simulink model "KalmanFilterBasic"  (R2020a)
settings: Solver=VariableStepAuto  StartTime=0.0  StopTime=10  RelTol=1e-3
PostLoadFcn:
  | cd 'C:\Users\rag\Documents\GitHub\EPQ\Rocket'
  | masscgI = xlsread('mass,cg,I','mass,cg,I');
  | ThrustTable = xlsread('F10_Thrust','Sheet1');
values from neighbouring files (symbols this model uses):
  D = zeros(size(B))    [RocketOutputFunction.m]    (also in StateSpaceController.m = zeros(13, 3); TimeDelayCompensationElevator.m = [0; 0])
undefined symbols (not defined in the file or in its folder): e0_0, e1_0, e2_0, e3_0
libraries: sharedTrackingLibrary x5, aerolibcommonsys x4, shared6dof x4, sharedtransform x3, shared6dofsys x2, dspmtrx3 x1, mspsensorlib x1, simulink x1, sharedutil x1, aerolibnav x1, dspstat3 x1
settings Model: Creator=rag  LastModifiedBy=rag
settings SFSimCC: CustomCodeUndefinedFunction=UseInterfaceOnly

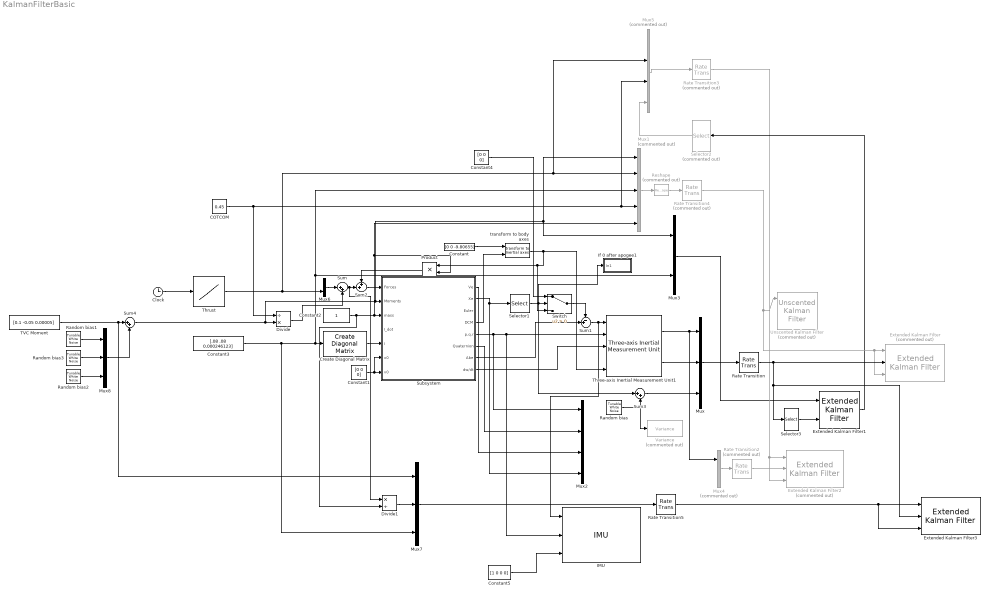
== system KalmanFilterBasic ==
  COTCOM : Constant  Value=0.45
  Clock : Clock
      settings: Decimation=100
  Constant : Constant  Value=[0 0 -9.80655]
  Constant1 : Constant  Value=[0 0 0]
  Constant2 : Constant
  Constant3 : Constant  Value=[.08 .08 0.000246123]
  Constant4 : Constant  Value=[0 0 0]
  Constant5 : Constant  Value=[1 0 0 0]
  Create Diagonal Matrix : dspmtrx3/Create Diagonal Matrix
      settings: SourceProductBaseCode=DS
  Divide : Product  Inputs=/*
  Divide1 : Product  Inputs=*/
  Extended Kalman Filter : sharedTrackingLibrary/Extended Kalman Filter  Commented=on  StateTransitionFcn=vdpStateFcn  HasStateTransitionJacobianFcn=off  HasAdditiveProcessNoise=Nonadditive  ProcessNoise=0.001 * eye(3)  HasTimeVaryingProcessNoise=off  HasStateTransitionFcnExtraArgument=1  InitialState=[zeros(1, 3) 1 zeros(1, 9)]  InitialStateCovariance=0.0000000001  MeasurementFcn1=vdpMeasurementNonAdditiveNoiseFcn  HasMeasurementJacobianFcn1=off  HasMeasurementEnablePort1=off  HasAdditiveMeasurementNoise1=Nonadditive  MeasurementNoise1=diag([0.001/0.001 0.001/0.001 0.001/0.001])  HasTimeVaryingMeasurementNoise1=off  HasMeasurementFcnExtraArgument1=1  MeasurementFcn2=myMeasurementFcn  HasMeasurementJacobianFcn2=off  HasMeasurementEnablePort2=off  HasAdditiveMeasurementNoise2=Additive  MeasurementNoise2=1  HasTimeVaryingMeasurementNoise2=off  HasMeasurementFcnExtraArgument2=0  MeasurementFcn3=myMeasurementFcn  HasMeasurementJacobianFcn3=off  HasMeasurementEnablePort3=off  HasAdditiveMeasurementNoise3=Additive  MeasurementNoise3=1  HasTimeVaryingMeasurementNoise3=off  HasMeasurementFcnExtraArgument3=0  MeasurementFcn4=myMeasurementFcn  HasMeasurementJacobianFcn4=off  HasMeasurementEnablePort4=off  HasAdditiveMeasurementNoise4=Additive  MeasurementNoise4=1  HasTimeVaryingMeasurementNoise4=off  HasMeasurementFcnExtraArgument4=0  MeasurementFcn5=myMeasurementFcn  HasMeasurementJacobianFcn5=off  HasMeasurementEnablePort5=off  HasAdditiveMeasurementNoise5=Additive  MeasurementNoise5=1  HasTimeVaryingMeasurementNoise5=off  HasMeasurementFcnExtraArgument5=0  EnableMultirate=off  StateTransitionFcnSampleTime=1  MeasurementFcn1SampleTime=1  MeasurementFcn2SampleTime=1  MeasurementFcn3SampleTime=1  MeasurementFcn4SampleTime=1  MeasurementFcn5SampleTime=1  UseCurrentEstimator=on  OutputStateCovariance=off  DataType=double  SampleTime=.2  NumberOfMeasurements=1
      settings: SourceProductBaseCode=CT,DR,TF,ID,NV,AR,RO,VE
  Extended Kalman Filter1 : sharedTrackingLibrary/Extended Kalman Filter  StateTransitionFcn=vdpStateFcnAttitudeOnly  HasStateTransitionJacobianFcn=off  HasAdditiveProcessNoise=Nonadditive  ProcessNoise=[1 1 0.001]  HasTimeVaryingProcessNoise=off  HasStateTransitionFcnExtraArgument=1  InitialState=[0 0 0 1 0 0 0]  InitialStateCovariance=1e-7  MeasurementFcn1=vdpMeasurementNonAdditiveNoiseFcnAttitudeOnly  HasMeasurementJacobianFcn1=off  HasMeasurementEnablePort1=off  HasAdditiveMeasurementNoise1=Nonadditive  MeasurementNoise1=1e-3 * eye(3)  HasTimeVaryingMeasurementNoise1=off  HasMeasurementFcnExtraArgument1=0  MeasurementFcn2=myMeasurementFcn  HasMeasurementJacobianFcn2=off  HasMeasurementEnablePort2=off  HasAdditiveMeasurementNoise2=Additive  MeasurementNoise2=1  HasTimeVaryingMeasurementNoise2=off  HasMeasurementFcnExtraArgument2=0  MeasurementFcn3=myMeasurementFcn  HasMeasurementJacobianFcn3=off  HasMeasurementEnablePort3=off  HasAdditiveMeasurementNoise3=Additive  MeasurementNoise3=1  HasTimeVaryingMeasurementNoise3=off  HasMeasurementFcnExtraArgument3=0  MeasurementFcn4=myMeasurementFcn  HasMeasurementJacobianFcn4=off  HasMeasurementEnablePort4=off  HasAdditiveMeasurementNoise4=Additive  MeasurementNoise4=1  HasTimeVaryingMeasurementNoise4=off  HasMeasurementFcnExtraArgument4=0  MeasurementFcn5=myMeasurementFcn  HasMeasurementJacobianFcn5=off  HasMeasurementEnablePort5=off  HasAdditiveMeasurementNoise5=Additive  MeasurementNoise5=1  HasTimeVaryingMeasurementNoise5=off  HasMeasurementFcnExtraArgument5=0  EnableMultirate=off  StateTransitionFcnSampleTime=1  MeasurementFcn1SampleTime=1  MeasurementFcn2SampleTime=1  MeasurementFcn3SampleTime=1  MeasurementFcn4SampleTime=1  MeasurementFcn5SampleTime=1  UseCurrentEstimator=on  OutputStateCovariance=off  DataType=double  SampleTime=0.001  NumberOfMeasurements=1
      settings: SourceProductBaseCode=CT,DR,TF,ID,NV,AR,RO,VE
  Extended Kalman Filter2 : sharedTrackingLibrary/Extended Kalman Filter  Commented=on  StateTransitionFcn=vdpStateFcnTranslationOnly  HasStateTransitionJacobianFcn=off  HasAdditiveProcessNoise=Nonadditive  ProcessNoise=0.001 * eye(3)  HasTimeVaryingProcessNoise=off  HasStateTransitionFcnExtraArgument=1  InitialState=[0 0 0 0 0 0]  InitialStateCovariance=1  MeasurementFcn1=vdpMeasurementNonAdditiveNoiseFcnTranslationOnly  HasMeasurementJacobianFcn1=off  HasMeasurementEnablePort1=off  HasAdditiveMeasurementNoise1=Nonadditive  MeasurementNoise1=diag([2 2 2 5])  HasTimeVaryingMeasurementNoise1=off  HasMeasurementFcnExtraArgument1=1  MeasurementFcn2=myMeasurementFcn  HasMeasurementJacobianFcn2=off  HasMeasurementEnablePort2=off  HasAdditiveMeasurementNoise2=Additive  MeasurementNoise2=1  HasTimeVaryingMeasurementNoise2=off  HasMeasurementFcnExtraArgument2=0  MeasurementFcn3=myMeasurementFcn  HasMeasurementJacobianFcn3=off  HasMeasurementEnablePort3=off  HasAdditiveMeasurementNoise3=Additive  MeasurementNoise3=1  HasTimeVaryingMeasurementNoise3=off  HasMeasurementFcnExtraArgument3=0  MeasurementFcn4=myMeasurementFcn  HasMeasurementJacobianFcn4=off  HasMeasurementEnablePort4=off  HasAdditiveMeasurementNoise4=Additive  MeasurementNoise4=1  HasTimeVaryingMeasurementNoise4=off  HasMeasurementFcnExtraArgument4=0  MeasurementFcn5=myMeasurementFcn  HasMeasurementJacobianFcn5=off  HasMeasurementEnablePort5=off  HasAdditiveMeasurementNoise5=Additive  MeasurementNoise5=1  HasTimeVaryingMeasurementNoise5=off  HasMeasurementFcnExtraArgument5=0  EnableMultirate=off  StateTransitionFcnSampleTime=1  MeasurementFcn1SampleTime=1  MeasurementFcn2SampleTime=1  MeasurementFcn3SampleTime=1  MeasurementFcn4SampleTime=1  MeasurementFcn5SampleTime=1  UseCurrentEstimator=on  OutputStateCovariance=off  DataType=double  SampleTime=0.001  NumberOfMeasurements=1
      settings: SourceProductBaseCode=CT,DR,TF,ID,NV,AR,RO,VE
  Extended Kalman Filter3 : sharedTrackingLibrary/Extended Kalman Filter  StateTransitionFcn=vdpStateFcn  HasStateTransitionJacobianFcn=off  HasAdditiveProcessNoise=Nonadditive  ProcessNoise=[.1 .1 1e-5]  HasTimeVaryingProcessNoise=off  HasStateTransitionFcnExtraArgument=1  InitialState=[zeros(1,3) 1 zeros(1,9)]  InitialStateCovariance=1e-9  MeasurementFcn1=vdpMeasurementNonAdditiveNoiseFcn  HasMeasurementJacobianFcn1=off  HasMeasurementEnablePort1=off  HasAdditiveMeasurementNoise1=Nonadditive  MeasurementNoise1=diag([.1 .1 .1 .1 .1 .1 1])  HasTimeVaryingMeasurementNoise1=off  HasMeasurementFcnExtraArgument1=1  MeasurementFcn2=myMeasurementFcn  HasMeasurementJacobianFcn2=off  HasMeasurementEnablePort2=off  HasAdditiveMeasurementNoise2=Additive  MeasurementNoise2=1  HasTimeVaryingMeasurementNoise2=off  HasMeasurementFcnExtraArgument2=0  MeasurementFcn3=myMeasurementFcn  HasMeasurementJacobianFcn3=off  HasMeasurementEnablePort3=off  HasAdditiveMeasurementNoise3=Additive  MeasurementNoise3=1  HasTimeVaryingMeasurementNoise3=off  HasMeasurementFcnExtraArgument3=0  MeasurementFcn4=myMeasurementFcn  HasMeasurementJacobianFcn4=off  HasMeasurementEnablePort4=off  HasAdditiveMeasurementNoise4=Additive  MeasurementNoise4=1  HasTimeVaryingMeasurementNoise4=off  HasMeasurementFcnExtraArgument4=0  MeasurementFcn5=myMeasurementFcn  HasMeasurementJacobianFcn5=off  HasMeasurementEnablePort5=off  HasAdditiveMeasurementNoise5=Additive  MeasurementNoise5=1  HasTimeVaryingMeasurementNoise5=off  HasMeasurementFcnExtraArgument5=0  EnableMultirate=off  StateTransitionFcnSampleTime=1  MeasurementFcn1SampleTime=1  MeasurementFcn2SampleTime=1  MeasurementFcn3SampleTime=1  MeasurementFcn4SampleTime=1  MeasurementFcn5SampleTime=1  UseCurrentEstimator=on  OutputStateCovariance=off  DataType=double  SampleTime=0.001  NumberOfMeasurements=1
      settings: SourceProductBaseCode=CT,DR,TF,ID,NV,AR,RO,VE
  IMU : mspsensorlib/IMU  DispRefFrame=NED  Temperature=25  MagneticFieldNED=[ 27.5550, -2.4169, -16.0849 ]  MagneticFieldENU=[ -2.4169, 27.5550, 16.0849 ]  SeedDouble=67  SimulateUsing=Interpreted execution  AccelParamsMeasurementRange=Inf  AccelParamsResolution=0  AccelParamsConstantBias=[ 0, 0, 0 ]  AccelParamsAxesMisalignment=[ 0, 0, 0 ]  AccelParamsNoiseDensity=[ 0, 0, 0 ]  AccelParamsBiasInstability=[ 0, 0, 0 ]  AccelParamsRandomWalk=[ 0, 0, 0 ]  AccelParamsTemperatureBias=[ 0, 0, 0 ]  AccelParamsTemperatureScaleFactor=[ 0, 0, 0 ]  GyroParamsMeasurementRange=Inf  GyroParamsResolution=0  GyroParamsConstantBias=[ 0, 0, 0 ]  GyroParamsAxesMisalignment=[ 0, 0, 0 ]  GyroParamsAccelerationBias=[ 0, 0, 0 ]  GyroParamsNoiseDensity=[ 0, 0, 0 ]  GyroParamsBiasInstability=[ 0, 0, 0 ]  GyroParamsRandomWalk=[ 0, 0, 0 ]  GyroParamsTemperatureBias=[ 0, 0, 0 ]  GyroParamsTemperatureScaleFactor=[ 0, 0, 0 ]  MagParamsMeasurementRange=Inf  MagParamsResolution=0  MagParamsConstantBias=[ 0, 0, 0 ]  MagParamsAxesMisalignment=[ 0, 0, 0 ]  MagParamsNoiseDensity=[ 0, 0, 0 ]  MagParamsBiasInstability=[ 0, 0, 0 ]  MagParamsRandomWalk=[ 0, 0, 0 ]  MagParamsTemperatureBias=[ 0, 0, 0 ]  MagParamsTemperatureScaleFactor=[ 0, 0, 0 ]
      settings: SourceProductBaseCode=TF,NV
  If 0 after apogee1 : Subsystem
  Mux{,6..8} (4 alike) : Mux  Inputs=3
  Mux1 : Mux  Commented=on  Inputs=5
  Mux2 : Mux
  Mux3 : Mux  Inputs=2
  Mux4 : Mux  Commented=on  Inputs=2
  Mux5 : Mux  Commented=on
  Product : Product
  Random bias : aerolibcommonsys/Tunable White Noise  pwr=0.001  Ts=0.001  seed=23341
      settings: SourceProductBaseCode=AE
  Random bias1 : aerolibcommonsys/Tunable White Noise  pwr=.1  Ts=1  seed=23341
      settings: SourceProductBaseCode=AE
  Random bias2 : aerolibcommonsys/Tunable White Noise  pwr=1e-8  Ts=0.001  seed=23341
      settings: SourceProductBaseCode=AE
  Random bias3 : aerolibcommonsys/Tunable White Noise  pwr=.1  Ts=1  seed=23341
      settings: SourceProductBaseCode=AE
  Rate Transition : RateTransition
  Rate Transition2 : RateTransition  Commented=on
  Rate Transition3 : RateTransition  Commented=on
  Rate Transition4 : RateTransition  Commented=on
  Rate Transition5 : RateTransition
  Reshape : Reshape  Commented=on  OutputDimensionality=Column vector (2-D)
  Selector1 : Selector  InputPortWidth=3  IndexOptions=Index vector (dialog)  Indices=3  OutputSizes=1
  Selector2 : Selector  Commented=on  InputPortWidth=7  IndexOptions=Index vector (dialog)  Indices=[4 5 6 7]  OutputSizes=1
  Selector3 : Selector  InputPortWidth=7  IndexOptions=Index vector (dialog)  Indices=1:3  OutputSizes=1
  Subsystem : Subsystem
  Sum : Sum  Inputs=|++
  Sum1 : Sum  Inputs=-+|
  Sum2 : Sum  Inputs=++|
  Sum3 : Sum  Inputs=|++
  Sum4 : Sum  Inputs=|++
  Switch : Switch  Criteria=u2 > Threshold
  TVC Moment : Constant  Value=[0.1 -0.05 0.00005]
  Three-axis Inertial Measurement Unit1 : aerolibnav/Three-axis Inertial Measurement Unit  units=Metric (MKS)  imu=[0 0 0]  i_Ts=0.001  dtype_a=off  w_a=190  z_a=0.707  a_sf_cc=[1 0 0; 0 1 0; 0 0 1]  a_bias=[0 0 0]  a_sat="[-inf  -inf  -inf  inf inf inf]"  dtype_g=off  w_g=190  z_g=0.707  g_sf_cc=[1 0 0; 0 1 0; 0 0 1]  g_bias=[0 0 0]  g_sens=[0 0 0]  g_sat="[-inf  -inf  -inf  inf inf inf]"  i_rand=on  i_seeds=[23093 23094 23095 23096 23097 23098]  i_pow=[0.0001 0.0001 0.0001 0.00001 0.00001 0.00001]
  Thrust : Lookup_n-D  NumberOfTableDimensions=1  BreakpointsForDimension1=ThrustTable(:,1)  BreakpointsForDimension1FirstPoint=0  BreakpointsForDimension1Spacing=1.5e-5  Table=ThrustTable(:,2)  ExtrapMethod=Clip  InternalRulePriority=Speed  RndMeth=Simplest  InputSameDT=on
  Unscented Kalman Filter : sharedTrackingLibrary/Unscented Kalman Filter  Commented=on  StateTransitionFcn=vdpStateFcn  HasAdditiveProcessNoise=Nonadditive  ProcessNoise=diag([3 3 .5 5 5 5])  HasTimeVaryingProcessNoise=off  HasStateTransitionFcnExtraArgument=1  InitialState=[zeros(1, 3) 1 zeros(1, 9)]  InitialStateCovariance=1  Alpha=1e-3  Beta=2  Kappa=0  MeasurementFcn1=vdpMeasurementNonAdditiveNoiseFcn  HasMeasurementEnablePort1=off  HasAdditiveMeasurementNoise1=Nonadditive  MeasurementNoise1=diag([1 1 .1 2 2 2 4])  HasTimeVaryingMeasurementNoise1=off  HasMeasurementFcnExtraArgument1=1  MeasurementFcn2=myMeasurementFcn  HasMeasurementEnablePort2=off  HasAdditiveMeasurementNoise2=Additive  MeasurementNoise2=1  HasTimeVaryingMeasurementNoise2=off  HasMeasurementFcnExtraArgument2=0  MeasurementFcn3=myMeasurementFcn  HasMeasurementEnablePort3=off  HasAdditiveMeasurementNoise3=Additive  MeasurementNoise3=1  HasTimeVaryingMeasurementNoise3=off  HasMeasurementFcnExtraArgument3=0  MeasurementFcn4=myMeasurementFcn  HasMeasurementEnablePort4=off  HasAdditiveMeasurementNoise4=Additive  MeasurementNoise4=1  HasTimeVaryingMeasurementNoise4=off  HasMeasurementFcnExtraArgument4=0  MeasurementFcn5=myMeasurementFcn  HasMeasurementEnablePort5=off  HasAdditiveMeasurementNoise5=Additive  MeasurementNoise5=1  HasTimeVaryingMeasurementNoise5=off  HasMeasurementFcnExtraArgument5=0  EnableMultirate=off  StateTransitionFcnSampleTime=1  MeasurementFcn1SampleTime=1  MeasurementFcn2SampleTime=1  MeasurementFcn3SampleTime=1  MeasurementFcn4SampleTime=1  MeasurementFcn5SampleTime=1  UseCurrentEstimator=on  OutputStateCovariance=off  DataType=double  SampleTime=0.0001  NumberOfMeasurements=1
      settings: SourceProductBaseCode=CT,DR,TF,ID,NV,AR,RO,VE
  Variance : dspstat3/Variance  Commented=on  run=on  InputProcessing=Columns as channels (frame based)  reset_popup=None  directionMode=Each column  dimension=1  roiEnable=off  roiType=Rectangles  roiPortion=Entire ROI  roiOutput=Individual statistics for each ROI  roiFlag=off  roundingMode=Floor  overflowMode=off
  "transform to body axes " : shared6dof/6DOF (Euler Angles)/transform to Inertial axes   SystemSampleTime=-1  Latency=0  AutoFrameSizeCalculation=off
      settings: SourceProductBaseCode=AE,PW,MT,VE,VP
  wires:
  Subsystem/2(Xe) -> Mux2/4, Selector1/1
  Selector1/1 -> Sum3/1, If 0 after apogee1/1(In1), Switch/2
  Three-axis Inertial Measurement Unit1/2 -> Mux/2
  Three-axis Inertial Measurement Unit1/1 -> Mux4/1, Mux/1
  Mux/1 -> Rate Transition/1
  Subsystem/7(Abe) -> Sum1/2
  Subsystem/5(p,q,r) -> IMU/2, Three-axis Inertial Measurement Unit1/2, Mux2/1
  Subsystem/8(dw/dt) -> Three-axis Inertial Measurement Unit1/3
  "transform to body axes "/1 -> Three-axis Inertial Measurement Unit1/5, Switch/3, Product/1
  Subsystem/4(DCM) -> "transform to body axes "/2
  Constant1/1 -> Subsystem/6(x0), Subsystem/7(v0)
  Constant2/1 -> Divide1/2, Product/2, Mux1/5, Subsystem/3(mass)
  Create Diagonal Matrix/1 -> Subsystem/5(I)
  Constant3/1 -> Mux7/3, Mux1/3, Mux3/2, Create Diagonal Matrix/1
  Sum/1 -> Divide1/1, Sum2/2
  COTCOM/1 -> Divide/1, Mux5/3, Mux1/4
  Mux1/1 -> Reshape/1
  Subsystem/6(Quaternion) -> Mux2/2
  Subsystem/1(Ve) -> Mux2/3
  Mux3/1 -> Extended Kalman Filter1/1
  Selector3/1 -> Extended Kalman Filter1/2
  Mux4/1 -> Rate Transition2/1
  Rate Transition2/1 -> Extended Kalman Filter2/2
  Mux5/1 -> Rate Transition3/1
  Rate Transition3/1 -> Extended Kalman Filter2/1, Extended Kalman Filter2/3
  Extended Kalman Filter1/1 -> Selector2/1
  Selector2/1 -> Mux5/4
  Thrust/1 -> Mux5/2, Mux1/2, Mux6/3
  Rate Transition4/1 -> Extended Kalman Filter/3, Extended Kalman Filter/1, Unscented Kalman Filter/1
  Constant/1 -> "transform to body axes "/1
  Constant4/1 -> Switch/1
  Product/1 -> Sum2/1
  Sum1/1 -> IMU/1, Three-axis Inertial Measurement Unit1/1
  Switch/1 -> Sum1/1
  Sum4/1 -> Divide/2, Subsystem/2(Moments), Mux3/1, Mux1/1
  Reshape/1 -> Rate Transition4/1
  Sum2/1 -> Subsystem/1(Forces)
  Mux6/1 -> Sum/1
  Divide/1 -> Sum/2
  Mux7/1 -> Rate Transition5/1
  Rate Transition5/1 -> Extended Kalman Filter3/3, Extended Kalman Filter3/1
  Rate Transition/1 -> Extended Kalman Filter/2, Selector3/1, Extended Kalman Filter3/2
  Random bias/1 -> Variance/1, Sum3/2
  Sum3/1 -> Mux/3
  Clock/1 -> Thrust/1
  Divide1/1 -> Mux7/2
  Mux8/1 -> Sum4/2
  Random bias1/1 -> Mux8/1
  Random bias2/1 -> Mux8/3
  Random bias3/1 -> Mux8/2
  TVC Moment/1 -> Mux7/1, Sum4/1
  Constant5/1 -> IMU/3

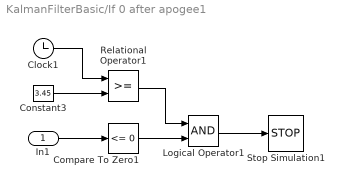
== system KalmanFilterBasic/If 0 after apogee1 ==
  In1 : Inport
  Clock1 : Clock
  Compare To Zero1 : simulink/Logic and Bit Operations/Compare To Zero  relop=<=  OutDataTypeStr=boolean
  Constant3 : Constant  Value=3.45
  Logical Operator1 : Logic  AllPortsSameDT=off  OutDataTypeStr=boolean
  Relational Operator1 : RelationalOperator  OutDataTypeStr=boolean  RndMeth=Simplest
  Stop Simulation1 : Stop
  wires:
  Clock1/1 -> Relational Operator1/1
  Constant3/1 -> Relational Operator1/2
  In1/1 -> Compare To Zero1/1
  Logical Operator1/1 -> Stop Simulation1/1
  Compare To Zero1/1 -> Logical Operator1/2
  Relational Operator1/1 -> Logical Operator1/1

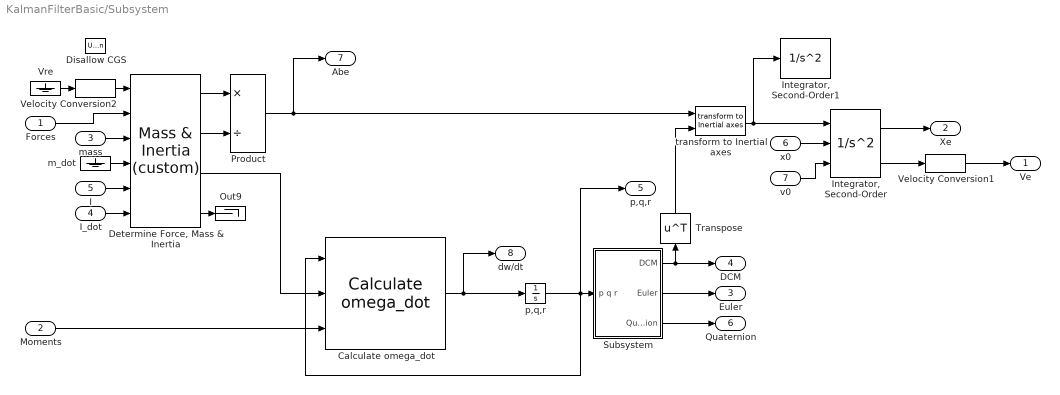
== system KalmanFilterBasic/Subsystem ==
  Forces : Inport  Unit=N  PortDimensions=3
  Moments : Inport  Port=2  Unit=N*m  PortDimensions=3
  mass : Inport  Port=3  Unit=kg
  I_dot : Inport  Port=4  Unit=kg*m^2/s  PortDimensions=[3 3]
  I : Inport  Port=5  Unit=kg*m^2  PortDimensions=[3 3]
  x0 : Inport  Port=6
  v0 : Inport  Port=7
  Calculate omega_dot : shared6dofsys/Calculate omega_dot  aMode=aMode
      settings: SourceProductBaseCode=AE,PW,MT,VE,VP
  "Determine Force, Mass & Inertia" : shared6dofsys/Mass & Inertia (custom)  aMode=aMode
      settings: SourceProductBaseCode=AE,PW,MT,VE,VP
  Disallow CGS : UnitConfiguration  UnitSystemsStr=English,SI,SI (extended)  AllowAllUnitSystems=off
  "Integrator, Second-Order" : SecondOrderIntegrator  ICSourceX=external  ICX=7.13*9.80655*3-(325.059163748137/mean(masscgI(:,2)) - .5 * 9.80655* 7.13^2)  LimitX=on  LowerLimitX=[-inf, -inf, 0]  ICSourceDXDT=external
  "Integrator, Second-Order1" : SecondOrderIntegrator  LimitX=on  LowerLimitX=[-inf, -inf, 0]
  Out9 : Terminator
  Product : Product  Inputs=*/  SaturateOnIntegerOverflow=on  OutDataTypeStr=Inherit: Same as first input
  Subsystem : Subsystem
  Transpose : Math  Operator=transpose  SignedPower=on  SaturateOnIntegerOverflow=on
  Velocity Conversion1 : shared6dof/6DOF (Euler Angles)/Velocity Conversion1  SystemSampleTime=-1  Latency=0  AutoFrameSizeCalculation=off
      settings: SourceProductBaseCode=AE,PW,MT,VE,VP
  Velocity Conversion2 : shared6dof/6DOF (Euler Angles)/Velocity Conversion2  SystemSampleTime=-1  Latency=0  AutoFrameSizeCalculation=off
      settings: SourceProductBaseCode=AE,PW,MT,VE,VP
  Vre : Ground
  m_dot : Ground
  "p,q,r " : Integrator  InitialCondition=[0 0 0]
  "transform to Inertial axes " : shared6dof/6DOF (Euler Angles)/transform to Inertial axes   SystemSampleTime=-1  Latency=0  AutoFrameSizeCalculation=off
      settings: SourceProductBaseCode=AE,PW,MT,VE,VP
  Ve : Outport  Unit=m/s  VectorParamsAs1DForOutWhenUnconnected=off
  Xe : Outport  Port=2  Unit=m  VectorParamsAs1DForOutWhenUnconnected=off
  Euler : Outport  Port=3  Unit=rad  VectorParamsAs1DForOutWhenUnconnected=off
  DCM : Outport  Port=4  Unit=1  VectorParamsAs1DForOutWhenUnconnected=off
  p,q,r : Outport  Port=5  Unit=rad/s  VectorParamsAs1DForOutWhenUnconnected=off
  Quaternion : Outport  Port=6  VectorParamsAs1DForOutWhenUnconnected=off
  Abe : Outport  Port=7  VectorParamsAs1DForOutWhenUnconnected=off
  dw/dt : Outport  Port=8  VectorParamsAs1DForOutWhenUnconnected=off
  wires:
  Subsystem/2(Euler) -> Euler/1
  "Determine Force, Mass & Inertia"/3 -> Calculate omega_dot/2
  "p,q,r "/1 -> Subsystem/1(p q r), p,q,r/1, Calculate omega_dot/1
  "transform to Inertial axes "/1 -> "Integrator, Second-Order1"/1, "Integrator, Second-Order"/1
  mass/1 -> "Determine Force, Mass & Inertia"/3
  Velocity Conversion1/1 -> Ve/1
  Subsystem/1(DCM) -> DCM/1, Transpose/1
  Calculate omega_dot/1 -> dw/dt/1, "p,q,r "/1
  Transpose/1 -> "transform to Inertial axes "/2
  Forces/1 -> "Determine Force, Mass & Inertia"/2
  "Determine Force, Mass & Inertia"/4 -> Out9/1
  I_dot/1 -> "Determine Force, Mass & Inertia"/6
  I/1 -> "Determine Force, Mass & Inertia"/5
  Velocity Conversion2/1 -> "Determine Force, Mass & Inertia"/1
  Vre/1 -> Velocity Conversion2/1
  "Determine Force, Mass & Inertia"/1 -> Product/1
  "Determine Force, Mass & Inertia"/2 -> Product/2
  m_dot/1 -> "Determine Force, Mass & Inertia"/4
  Subsystem/3(Quaternion) -> Quaternion/1
  Moments/1 -> Calculate omega_dot/3
  "Integrator, Second-Order"/2 -> Velocity Conversion1/1
  "Integrator, Second-Order"/1 -> Xe/1
  Product/1 -> Abe/1, "transform to Inertial axes "/1
  v0/1 -> "Integrator, Second-Order"/3
  x0/1 -> "Integrator, Second-Order"/2

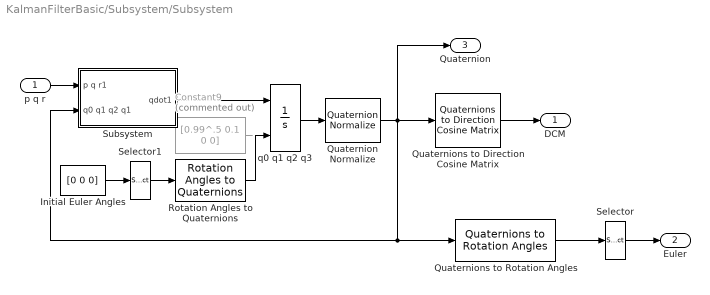
== system KalmanFilterBasic/Subsystem/Subsystem ==
  p q r : Inport
  Constant9 : Constant  Commented=on  Value=[0.99^.5 0.1 0 0]
  Initial Euler Angles : Constant  Value=[0 0 0]
  Quaternion Normalize : sharedutil/Quaternion Normalize  aMode=aMode
      settings: SourceProductBaseCode=AE,PW,MT,VE,VP
  Quaternions to Direction Cosine Matrix : sharedtransform/Quaternions to  Direction Cosine Matrix  aMode=aMode
      settings: SourceProductBaseCode=AE,PW,MT,VE,VP
  Quaternions to Rotation Angles : sharedtransform/Quaternions to Rotation Angles  rotationOrder=ZYX  aMode=aMode
      settings: SourceProductBaseCode=AE,PW,MT,VE,VP
  Rotation Angles to Quaternions : sharedtransform/Rotation Angles to Quaternions  rotationOrder=ZYX  aMode=aMode
      settings: SourceProductBaseCode=AE,PW,MT,VE,VP
  Selector : Selector  IndexMode=Zero-based  InputPortWidth=3  IndexOptions=Index vector (dialog)  Indices=[ 2 1 0]  OutputSizes=1
  Selector1 : Selector  IndexMode=Zero-based  InputPortWidth=3  IndexOptions=Index vector (dialog)  Indices=[2 1 0]  OutputSizes=1
  Subsystem : Subsystem
  q0 q1 q2 q3 : Integrator  InitialConditionSource=external  InitialCondition=[e0_0 e1_0 e2_0 e3_0]
  DCM : Outport  VectorParamsAs1DForOutWhenUnconnected=off
  Euler : Outport  Port=2  VectorParamsAs1DForOutWhenUnconnected=off
  Quaternion : Outport  Port=3  VectorParamsAs1DForOutWhenUnconnected=off
  wires:
  Selector/1 -> Euler/1
  Initial Euler Angles/1 -> Selector1/1
  Selector1/1 -> Rotation Angles to Quaternions/1
  q0 q1 q2 q3/1 -> Quaternion Normalize/1
  Quaternions to Direction Cosine Matrix/1 -> DCM/1
  Subsystem/1(qdot1) -> q0 q1 q2 q3/1
  p q r/1 -> Subsystem/1(p q r1)
  Quaternions to Rotation Angles/1 -> Selector/1
  Quaternion Normalize/1 -> Quaternion/1, Subsystem/2(q0 q1 q2 q1), Quaternions to Rotation Angles/1, Quaternions to Direction Cosine Matrix/1
  Rotation Angles to Quaternions/1 -> q0 q1 q2 q3/2
  Constant9/1 -> ?

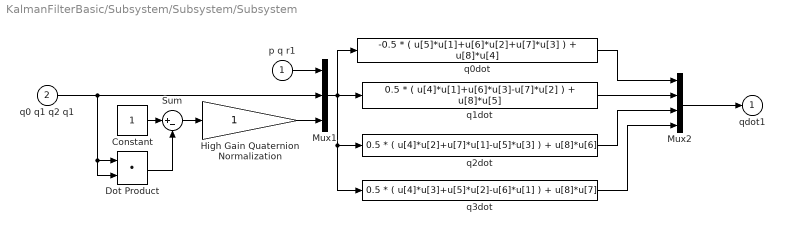
== system KalmanFilterBasic/Subsystem/Subsystem/Subsystem ==
  p q r1 : Inport
  q0 q1 q2 q1 : Inport  Port=2
  Constant : Constant
  Dot Product : DotProduct  OutDataTypeStr=Inherit: Inherit via internal rule
  High Gain Quaternion Normalization : Gain  SaturateOnIntegerOverflow=on  OutDataTypeStr=Inherit: Same as input  ParamDataTypeStr=Inherit: Same as input
  Mux1 : Mux  Inputs=[3 4 1]
  Mux2 : Mux
  Sum : Sum  Inputs=|+-  InputSameDT=on  SaturateOnIntegerOverflow=on  OutDataTypeStr=Inherit: Same as first input
  q0dot : Fcn  Expr=-0.5 * ( u[5]*u[1]+u[6]*u[2]+u[7]*u[3] ) + u[8]*u[4]
  q1dot : Fcn  Expr=0.5 * ( u[4]*u[1]+u[6]*u[3]-u[7]*u[2] ) + u[8]*u[5]
  q2dot : Fcn  Expr=0.5 * ( u[4]*u[2]+u[7]*u[1]-u[5]*u[3] ) + u[8]*u[6]
  q3dot : Fcn  Expr=0.5 * ( u[4]*u[3]+u[5]*u[2]-u[6]*u[1] ) + u[8]*u[7]
  qdot1 : Outport  InitialOutput=0  VectorParamsAs1DForOutWhenUnconnected=off
  wires:
  Constant/1 -> Sum/1
  Dot Product/1 -> Sum/2
  Mux1/1 -> q2dot/1, q3dot/1, q0dot/1, q1dot/1
  q0 q1 q2 q1/1 -> Dot Product/1, Dot Product/2, Mux1/2
  Sum/1 -> High Gain Quaternion Normalization/1
  Mux2/1 -> qdot1/1
  q0dot/1 -> Mux2/1
  q3dot/1 -> Mux2/4
  q1dot/1 -> Mux2/2
  q2dot/1 -> Mux2/3
  High Gain Quaternion Normalization/1 -> Mux1/3
  p q r1/1 -> Mux1/1
